simulink model "NarwhaleSimscape"  (R2021b)
settings: Solver=VariableStepAuto  StartTime=0.0  StopTime=12  FixedStep=10^-3  RelTol=1e-3
undefined symbols (not defined in the file): X, Y, Z
libraries: nesl_utility x34, sm_lib x28, slpidlib x5
(part 3 of 3)

== matlab function NarwhaleSimscape/NarWhale/IVK_5chi_dot ==
  data: q input; qv output; chi_dot input
function qv = IVK(q,chi_dot) %q,qv5,chi_dot  % q,taskspace
% h1= 275.99/1000; % lasted
% h2= 380/1000;
% l1= 20.01/1000;
% l2= 380/1000;
% l3= 235/1000;
% h1= 275.99/1000; % lasted
h2= 380/1000;
l1= 20/1000;
l2= 380/1000;
l3= 268.23/1000;

% qv = [                                                                                                                                                                                                                                                                                                                                                                                                                                                                                                                                                                                                                                                                                                                                                                                                                                                                                                                                                                                                                                                                                                                                                                                                                                                                                                                                                                                                                                                                                                                                                                                                                                                                                                                                                                                                                                                                                                                                                                                                                                                                                                                                                                                                                                                                                                                                                                                                                                                                                                                                                                                                                                                                                                                                                                                                                                                                                                                                                                                                                                                                                                                                                                                                                                                                                                                                                                                                                                                                                                                                                                                                                                                                                                                                                                                                                                                                                                                                                                                                                                                                                                                                                                                                                                                                                                                                                                                                                                                                                                                                                                                                                                                                                                                                                                                                                                                                                                                                                                                                                                                                                                                                                                                                                                                                                                                                                                                                                                                                                                                                                                                                                                                                                                                                                                                                                                                                                                                                                                                                                                                                                                                                                                                                                                                                                                                                                                                                                                                                                                                                                                                                                                                                                       (taskspace(4)*cos(q(1)) - taskspace(3)*sin(q(1)))/(l1 + l2*cos(q(2) + q(3)) - 1.0*h2*sin(q(2)) + l3*sin(q(2) + q(3) + q(4)));
%                                                                                                                                                                                                                                                                                                                                                                                                                                                                                                                                                                                                                                                                                                                                                                                                                                                                                                                                                                                                                                                                                                                                                                                                                                                                                                                                                                                                                                                                                                                                                                                                                                                                                                                                                                                                                                                                                                                                                                                                                                                                                                                                                                                                                                                                                                                                                                                                                                                                                                                                                                                                                                                                                                                                                                                                                                                                                                                                                                                                                                                                                                                                                                     -(1.0*(l3^2*taskspace(2)*sin(q(2) + q(3) + q(4))^3*sin(q(2) + q(3))*sin(q(1))^3 + l1*taskspace(3)*cos(q(2) + q(3) + q(4))*cos(q(2) + q(3))*cos(q(1))^2 + l1*taskspace(5)*cos(q(2) + q(3) + q(4))*sin(q(2) + q(3))*cos(q(1))^3 + l2*taskspace(3)*cos(q(2) + q(3) + q(4))*cos(q(2) + q(3))^2*cos(q(1))^2 + l3*taskspace(3)*sin(q(2) + q(3) + q(4))^2*sin(q(2) + q(3))*sin(q(1))^2 + l1*l3*taskspace(1)*cos(q(2) + q(3) + q(4))^2*cos(q(2) + q(3))*sin(q(1))^2 - h2*taskspace(3)*cos(q(2) + q(3) + q(4))*cos(q(2) + q(3))*cos(q(1))^2*sin(q(2)) + l2*taskspace(4)*cos(q(2) + q(3) + q(4))*cos(q(2) + q(3))^2*cos(q(1))*sin(q(1)) + l3^2*taskspace(1)*cos(q(2) + q(3) + q(4))^2*sin(q(2) + q(3) + q(4))*cos(q(2) + q(3))*cos(q(1))^2 - h2*taskspace(5)*cos(q(2) + q(3) + q(4))*sin(q(2) + q(3))*cos(q(1))^3*sin(q(2)) + l1*taskspace(5)*cos(q(2) + q(3) + q(4))*sin(q(2) + q(3))*cos(q(1))*sin(q(1))^2 + l3^2*taskspace(1)*cos(q(2) + q(3) + q(4))*sin(q(2) + q(3) + q(4))^2*sin(q(2) + q(3))*cos(q(1))^2 + l3^2*taskspace(1)*cos(q(2) + q(3) + q(4))^2*sin(q(2) + q(3) + q(4))*cos(q(2) + q(3))*sin(q(1))^2 + l3^2*taskspace(2)*cos(q(2) + q(3) + q(4))*sin(q(2) + q(3) + q(4))^2*cos(q(2) + q(3))*sin(q(1))^3 + l1*l3*taskspace(2)*sin(q(2) + q(3) + q(4))^2*sin(q(2) + q(3))*sin(q(1))^3 - l3*taskspace(4)*sin(q(2) + q(3) + q(4))^2*sin(q(2) + q(3))*cos(q(1))*sin(q(1)) + l3^2*taskspace(1)*cos(q(2) + q(3) + q(4))*sin(q(2) + q(3) + q(4))^2*sin(q(2) + q(3))*sin(q(1))^2 + l3*taskspace(3)*cos(q(2) + q(3) + q(4))*sin(q(2) + q(3) + q(4))*cos(q(2) + q(3))*cos(q(1))^2 + l2*l3*taskspace(1)*cos(q(2) + q(3) + q(4))^2*cos(q(2) + q(3))^2*cos(q(1))^2 + l3*taskspace(3)*cos(q(2) + q(3) + q(4))*sin(q(2) + q(3) + q(4))*cos(q(2) + q(3))*sin(q(1))^2 + l3*taskspace(5)*cos(q(2) + q(3) + q(4))*sin(q(2) + q(3) + q(4))*sin(q(2) + q(3))*cos(q(1))^3 + l2*l3*taskspace(1)*cos(q(2) + q(3) + q(4))^2*cos(q(2) + q(3))^2*sin(q(1))^2 + l1*taskspace(4)*cos(q(2) + q(3) + q(4))*cos(q(2) + q(3))*cos(q(1))*sin(q(1)) + l2*taskspace(5)*cos(q(2) + q(3) + q(4))*cos(q(2) + q(3))*sin(q(2) + q(3))*cos(q(1))^3 + l3^2*taskspace(2)*sin(q(2) + q(3) + q(4))^3*sin(q(2) + q(3))*cos(q(1))^2*sin(q(1)) + l1*l3*taskspace(1)*cos(q(2) + q(3) + q(4))^2*cos(q(2) + q(3))*cos(q(1))^2 + l1*l3*taskspace(2)*sin(q(2) + q(3) + q(4))^2*sin(q(2) + q(3))*cos(q(1))^2*sin(q(1)) - h2*taskspace(5)*cos(q(2) + q(3) + q(4))*sin(q(2) + q(3))*cos(q(1))*sin(q(1))^2*sin(q(2)) - h2*l3*taskspace(2)*sin(q(2) + q(3) + q(4))^2*sin(q(2) + q(3))*sin(q(1))^3*sin(q(2)) + l2*l3*taskspace(2)*cos(q(2) + q(3) + q(4))*sin(q(2) + q(3) + q(4))*cos(q(2) + q(3))^2*sin(q(1))^3 + l3*taskspace(5)*cos(q(2) + q(3) + q(4))*sin(q(2) + q(3) + q(4))*sin(q(2) + q(3))*cos(q(1))*sin(q(1))^2 - h2*taskspace(4)*cos(q(2) + q(3) + q(4))*cos(q(2) + q(3))*cos(q(1))*sin(q(1))*sin(q(2)) + l2*taskspace(5)*cos(q(2) + q(3) + q(4))*cos(q(2) + q(3))*sin(q(2) + q(3))*cos(q(1))*sin(q(1))^2 + l2*l3*taskspace(2)*sin(q(2) + q(3) + q(4))^2*cos(q(2) + q(3))*sin(q(2) + q(3))*sin(q(1))^3 + l1*l3*taskspace(1)*cos(q(2) + q(3) + q(4))*sin(q(2) + q(3) + q(4))*sin(q(2) + q(3))*cos(q(1))^2 + l1*l3*taskspace(2)*cos(q(2) + q(3) + q(4))*sin(q(2) + q(3) + q(4))*cos(q(2) + q(3))*sin(q(1))^3 - h2*l3*taskspace(1)*cos(q(2) + q(3) + q(4))^2*cos(q(2) + q(3))*cos(q(1))^2*sin(q(2)) + l1*l3*taskspace(1)*cos(q(2) + q(3) + q(4))*sin(q(2) + q(3) + q(4))*sin(q(2) + q(3))*sin(q(1))^2 - h2*l3*taskspace(1)*cos(q(2) + q(3) + q(4))^2*cos(q(2) + q(3))*sin(q(1))^2*sin(q(2)) + l3^2*taskspace(2)*cos(q(2) + q(3) + q(4))*sin(q(2) + q(3) + q(4))^2*cos(q(2) + q(3))*cos(q(1))^2*sin(q(1)) + l2*l3*taskspace(2)*cos(q(2) + q(3) + q(4))*sin(q(2) + q(3) + q(4))*cos(q(2) + q(3))^2*cos(q(1))^2*sin(q(1)) + l2*l3*taskspace(1)*cos(q(2) + q(3) + q(4))*sin(q(2) + q(3) + q(4))*cos(q(2) + q(3))*sin(q(2) + q(3))*cos(q(1))^2 + l2*l3*taskspace(1)*cos(q(2) + q(3) + q(4))*sin(q(2) + q(3) + q(4))*cos(q(2) + q(3))*sin(q(2) + q(3))*sin(q(1))^2 + l2*l3*taskspace(2)*sin(q(2) + q(3) + q(4))^2*cos(q(2) + q(3))*sin(q(2) + q(3))*cos(q(1))^2*sin(q(1)) + l1*l3*taskspace(2)*cos(q(2) + q(3) + q(4))*sin(q(2) + q(3) + q(4))*cos(q(2) + q(3))*cos(q(1))^2*sin(q(1)) - h2*l3*taskspace(1)*cos(q(2) + q(3) + q(4))*sin(q(2) + q(3) + q(4))*sin(q(2) + q(3))*cos(q(1))^2*sin(q(2)) - h2*l3*taskspace(2)*cos(q(2) + q(3) + q(4))*sin(q(2) + q(3) + q(4))*cos(q(2) + q(3))*sin(q(1))^3*sin(q(2)) - h2*l3*taskspace(1)*cos(q(2) + q(3) + q(4))*sin(q(2) + q(3) + q(4))*sin(q(2) + q(3))*sin(q(1))^2*sin(q(2)) - h2*l3*taskspace(2)*sin(q(2) + q(3) + q(4))^2*sin(q(2) + q(3))*cos(q(1))^2*sin(q(1))*sin(q(2)) - h2*l3*taskspace(2)*cos(q(2) + q(3) + q(4))*sin(q(2) + q(3) + q(4))*cos(q(2) + q(3))*cos(q(1))^2*sin(q(1))*sin(q(2))))/(h2*cos(q(1))*cos(q(3))*(0.5*l3*sin(2*q(2) + 2*q(3) + 2*q(4)) + 0.5*l2*cos(2.0*q(2) + 2.0*q(3) + q(4)) + 0.5*h2*sin(q(3) + q(4)) - 0.5*h2*sin(2.0*q(2) + q(3) + q(4)) + 0.5*l2*cos(q(4)) + l1*cos(q(2) + q(3) + q(4))));
% (1.0*(h2^2*taskspace(3)*cos(q(2) + q(3) + q(4))*cos(q(1))^2*sin(q(2))^2 + l2^2*taskspace(3)*cos(q(2) + q(3) + q(4))*cos(q(2) + q(3))^2*cos(q(1))^2 + h2^2*l3*taskspace(1)*cos(q(2) + q(3) + q(4))^2*sin(q(1))^2*sin(q(2))^2 + l2*l3*taskspace(3)*sin(q(2) + q(3) + q(4))^2*sin(q(2) + q(3))*sin(q(1))^2 + l2^2*taskspace(5)*cos(q(2) + q(3) + q(4))*cos(q(2) + q(3))*sin(q(2) + q(3))*cos(q(1))^3 + h2*l3*taskspace(3)*sin(q(2) + q(3) + q(4))^2*cos(q(2))*sin(q(1))^2 + l2^2*taskspace(4)*cos(q(2) + q(3) + q(4))*cos(q(2) + q(3))^2*cos(q(1))*sin(q(1)) + l2*l3^2*taskspace(2)*sin(q(2) + q(3) + q(4))^3*sin(q(2) + q(3))*sin(q(1))^3 + l1*l2*taskspace(3)*cos(q(2) + q(3) + q(4))*cos(q(2) + q(3))*cos(q(1))^2 - 1.0*h2^2*taskspace(5)*cos(q(2) + q(3) + q(4))*cos(q(1))^3*cos(q(2))*sin(q(2)) + h2*l3^2*taskspace(2)*sin(q(2) + q(3) + q(4))^3*cos(q(2))*sin(q(1))^3 + l1*l2*taskspace(5)*cos(q(2) + q(3) + q(4))*sin(q(2) + q(3))*cos(q(1))^3 + h2^2*taskspace(4)*cos(q(2) + q(3) + q(4))*cos(q(1))*sin(q(1))*sin(q(2))^2 + l2^2*l3*taskspace(1)*cos(q(2) + q(3) + q(4))^2*cos(q(2) + q(3))^2*cos(q(1))^2 + h2*l1*taskspace(5)*cos(q(2) + q(3) + q(4))*cos(q(1))^3*cos(q(2)) + l2^2*l3*taskspace(1)*cos(q(2) + q(3) + q(4))^2*cos(q(2) + q(3))^2*sin(q(1))^2 - 1.0*h2*l1*taskspace(3)*cos(q(2) + q(3) + q(4))*cos(q(1))^2*sin(q(2)) + h2^2*l3*taskspace(1)*cos(q(2) + q(3) + q(4))^2*cos(q(1))^2*sin(q(2))^2 - 1.0*h2*l3*taskspace(3)*cos(q(2) + q(3) + q(4))*sin(q(2) + q(3) + q(4))*sin(q(1))^2*sin(q(2)) + l1*l2*taskspace(4)*cos(q(2) + q(3) + q(4))*cos(q(2) + q(3))*cos(q(1))*sin(q(1)) + l2^2*taskspace(5)*cos(q(2) + q(3) + q(4))*cos(q(2) + q(3))*sin(q(2) + q(3))*cos(q(1))*sin(q(1))^2 + l2^2*l3*taskspace(2)*sin(q(2) + q(3) + q(4))^2*cos(q(2) + q(3))*sin(q(2) + q(3))*sin(q(1))^3 - 1.0*h2*l1*taskspace(4)*cos(q(2) + q(3) + q(4))*cos(q(1))*sin(q(1))*sin(q(2)) + l2*l3^2*taskspace(2)*sin(q(2) + q(3) + q(4))^3*sin(q(2) + q(3))*cos(q(1))^2*sin(q(1)) + l1*l2*l3*taskspace(1)*cos(q(2) + q(3) + q(4))^2*cos(q(2) + q(3))*cos(q(1))^2 + h2*l2*taskspace(5)*cos(q(2) + q(3) + q(4))*cos(q(2) + q(3))*cos(q(1))^3*cos(q(2)) + l1*l2*l3*taskspace(1)*cos(q(2) + q(3) + q(4))^2*cos(q(2) + q(3))*sin(q(1))^2 + h2*l3^2*taskspace(2)*sin(q(2) + q(3) + q(4))^3*cos(q(1))^2*cos(q(2))*sin(q(1)) - 2.0*h2*l2*taskspace(3)*cos(q(2) + q(3) + q(4))*cos(q(2) + q(3))*cos(q(1))^2*sin(q(2)) + l2*l3^2*taskspace(1)*cos(q(2) + q(3) + q(4))^2*sin(q(2) + q(3) + q(4))*cos(q(2) + q(3))*cos(q(1))^2 - 1.0*h2^2*taskspace(5)*cos(q(2) + q(3) + q(4))*cos(q(1))*cos(q(2))*sin(q(1))^2*sin(q(2)) - 1.0*h2^2*l3*taskspace(2)*sin(q(2) + q(3) + q(4))^2*cos(q(2))*sin(q(1))^3*sin(q(2)) - 1.0*h2*l2*taskspace(5)*cos(q(2) + q(3) + q(4))*sin(q(2) + q(3))*cos(q(1))^3*sin(q(2)) + l1*l2*taskspace(5)*cos(q(2) + q(3) + q(4))*sin(q(2) + q(3))*cos(q(1))*sin(q(1))^2 + l2*l3^2*taskspace(1)*cos(q(2) + q(3) + q(4))*sin(q(2) + q(3) + q(4))^2*sin(q(2) + q(3))*cos(q(1))^2 + l2*l3^2*taskspace(1)*cos(q(2) + q(3) + q(4))^2*sin(q(2) + q(3) + q(4))*cos(q(2) + q(3))*sin(q(1))^2 + l2*l3^2*taskspace(2)*cos(q(2) + q(3) + q(4))*sin(q(2) + q(3) + q(4))^2*cos(q(2) + q(3))*sin(q(1))^3 + l2^2*l3*taskspace(2)*cos(q(2) + q(3) + q(4))*sin(q(2) + q(3) + q(4))*cos(q(2) + q(3))^2*sin(q(1))^3 + l1*l2*l3*taskspace(2)*sin(q(2) + q(3) + q(4))^2*sin(q(2) + q(3))*sin(q(1))^3 - 1.0*l2*l3*taskspace(4)*sin(q(2) + q(3) + q(4))^2*sin(q(2) + q(3))*cos(q(1))*sin(q(1)) + l2*l3^2*taskspace(1)*cos(q(2) + q(3) + q(4))*sin(q(2) + q(3) + q(4))^2*sin(q(2) + q(3))*sin(q(1))^2 - 1.0*h2*l1*l3*taskspace(1)*cos(q(2) + q(3) + q(4))^2*cos(q(1))^2*sin(q(2)) + h2*l1*taskspace(5)*cos(q(2) + q(3) + q(4))*cos(q(1))*cos(q(2))*sin(q(1))^2 + h2*l3^2*taskspace(1)*cos(q(2) + q(3) + q(4))*sin(q(2) + q(3) + q(4))^2*cos(q(1))^2*cos(q(2)) - 1.0*h2*l1*l3*taskspace(1)*cos(q(2) + q(3) + q(4))^2*sin(q(1))^2*sin(q(2)) + h2*l1*l3*taskspace(2)*sin(q(2) + q(3) + q(4))^2*cos(q(2))*sin(q(1))^3 - 1.0*h2*l3*taskspace(4)*sin(q(2) + q(3) + q(4))^2*cos(q(1))*cos(q(2))*sin(q(1)) + h2*l3^2*taskspace(1)*cos(q(2) + q(3) + q(4))*sin(q(2) + q(3) + q(4))^2*cos(q(2))*sin(q(1))^2 - 1.0*h2*l3^2*taskspace(1)*cos(q(2) + q(3) + q(4))^2*sin(q(2) + q(3) + q(4))*cos(q(1))^2*sin(q(2)) + l2*l3*taskspace(3)*cos(q(2) + q(3) + q(4))*sin(q(2) + q(3) + q(4))*cos(q(2) + q(3))*cos(q(1))^2 - 1.0*h2*l3^2*taskspace(1)*cos(q(2) + q(3) + q(4))^2*sin(q(2) + q(3) + q(4))*sin(q(1))^2*sin(q(2)) - 1.0*h2*l3^2*taskspace(2)*cos(q(2) + q(3) + q(4))*sin(q(2) + q(3) + q(4))^2*sin(q(1))^3*sin(q(2)) + h2^2*l3*taskspace(2)*cos(q(2) + q(3) + q(4))*sin(q(2) + q(3) + q(4))*sin(q(1))^3*sin(q(2))^2 + l2*l3*taskspace(3)*cos(q(2) + q(3) + q(4))*sin(q(2) + q(3) + q(4))*cos(q(2) + q(3))*sin(q(1))^2 + l2*l3*taskspace(5)*cos(q(2) + q(3) + q(4))*sin(q(2) + q(3) + q(4))*sin(q(2) + q(3))*cos(q(1))^3 + h2*l3*taskspace(5)*cos(q(2) + q(3) + q(4))*sin(q(2) + q(3) + q(4))*cos(q(1))^3*cos(q(2)) - 1.0*h2*l3*taskspace(3)*cos(q(2) + q(3) + q(4))*sin(q(2) + q(3) + q(4))*cos(q(1))^2*sin(q(2)) - 2.0*h2*l2*taskspace(4)*cos(q(2) + q(3) + q(4))*cos(q(2) + q(3))*cos(q(1))*sin(q(1))*sin(q(2)) + l2^2*l3*taskspace(2)*sin(q(2) + q(3) + q(4))^2*cos(q(2) + q(3))*sin(q(2) + q(3))*cos(q(1))^2*sin(q(1)) - 1.0*h2^2*l3*taskspace(1)*cos(q(2) + q(3) + q(4))*sin(q(2) + q(3) + q(4))*cos(q(1))^2*cos(q(2))*sin(q(2)) + l1*l2*l3*taskspace(1)*cos(q(2) + q(3) + q(4))*sin(q(2) + q(3) + q(4))*sin(q(2) + q(3))*cos(q(1))^2 + l1*l2*l3*taskspace(2)*cos(q(2) + q(3) + q(4))*sin(q(2) + q(3) + q(4))*cos(q(2) + q(3))*sin(q(1))^3 - 1.0*h2^2*l3*taskspace(1)*cos(q(2) + q(3) + q(4))*sin(q(2) + q(3) + q(4))*cos(q(2))*sin(q(1))^2*sin(q(2)) - 2.0*h2*l2*l3*taskspace(1)*cos(q(2) + q(3) + q(4))^2*cos(q(2) + q(3))*cos(q(1))^2*sin(q(2)) + l1*l2*l3*taskspace(1)*cos(q(2) + q(3) + q(4))*sin(q(2) + q(3) + q(4))*sin(q(2) + q(3))*sin(q(1))^2 + h2*l2*taskspace(5)*cos(q(2) + q(3) + q(4))*cos(q(2) + q(3))*cos(q(1))*cos(q(2))*sin(q(1))^2 - 2.0*h2*l2*l3*taskspace(1)*cos(q(2) + q(3) + q(4))^2*cos(q(2) + q(3))*sin(q(1))^2*sin(q(2)) + h2*l2*l3*taskspace(2)*sin(q(2) + q(3) + q(4))^2*cos(q(2) + q(3))*cos(q(2))*sin(q(1))^3 + h2*l1*l3*taskspace(1)*cos(q(2) + q(3) + q(4))*sin(q(2) + q(3) + q(4))*cos(q(1))^2*cos(q(2)) - 1.0*h2^2*l3*taskspace(2)*sin(q(2) + q(3) + q(4))^2*cos(q(1))^2*cos(q(2))*sin(q(1))*sin(q(2)) + l2*l3^2*taskspace(2)*cos(q(2) + q(3) + q(4))*sin(q(2) + q(3) + q(4))^2*cos(q(2) + q(3))*cos(q(1))^2*sin(q(1)) + l2^2*l3*taskspace(2)*cos(q(2) + q(3) + q(4))*sin(q(2) + q(3) + q(4))*cos(q(2) + q(3))^2*cos(q(1))^2*sin(q(1)) + h2*l1*l3*taskspace(1)*cos(q(2) + q(3) + q(4))*sin(q(2) + q(3) + q(4))*cos(q(2))*sin(q(1))^2 + l1*l2*l3*taskspace(2)*sin(q(2) + q(3) + q(4))^2*sin(q(2) + q(3))*cos(q(1))^2*sin(q(1)) - 1.0*h2*l2*taskspace(5)*cos(q(2) + q(3) + q(4))*sin(q(2) + q(3))*cos(q(1))*sin(q(1))^2*sin(q(2)) - 1.0*h2*l2*l3*taskspace(2)*sin(q(2) + q(3) + q(4))^2*sin(q(2) + q(3))*sin(q(1))^3*sin(q(2)) - 1.0*h2*l1*l3*taskspace(2)*cos(q(2) + q(3) + q(4))*sin(q(2) + q(3) + q(4))*sin(q(1))^3*sin(q(2)) + h2*l1*l3*taskspace(2)*sin(q(2) + q(3) + q(4))^2*cos(q(1))^2*cos(q(2))*sin(q(1)) - 1.0*h2*l3^2*taskspace(2)*cos(q(2) + q(3) + q(4))*sin(q(2) + q(3) + q(4))^2*cos(q(1))^2*sin(q(1))*sin(q(2)) + h2^2*l3*taskspace(2)*cos(q(2) + q(3) + q(4))*sin(q(2) + q(3) + q(4))*cos(q(1))^2*sin(q(1))*sin(q(2))^2 + l2*l3*taskspace(5)*cos(q(2) + q(3) + q(4))*sin(q(2) + q(3) + q(4))*sin(q(2) + q(3))*cos(q(1))*sin(q(1))^2 + h2*l3*taskspace(5)*cos(q(2) + q(3) + q(4))*sin(q(2) + q(3) + q(4))*cos(q(1))*cos(q(2))*sin(q(1))^2 + l2^2*l3*taskspace(1)*cos(q(2) + q(3) + q(4))*sin(q(2) + q(3) + q(4))*cos(q(2) + q(3))*sin(q(2) + q(3))*cos(q(1))^2 + l2^2*l3*taskspace(1)*cos(q(2) + q(3) + q(4))*sin(q(2) + q(3) + q(4))*cos(q(2) + q(3))*sin(q(2) + q(3))*sin(q(1))^2 + h2*l2*l3*taskspace(1)*cos(q(2) + q(3) + q(4))*sin(q(2) + q(3) + q(4))*cos(q(2) + q(3))*cos(q(2))*sin(q(1))^2 + l1*l2*l3*taskspace(2)*cos(q(2) + q(3) + q(4))*sin(q(2) + q(3) + q(4))*cos(q(2) + q(3))*cos(q(1))^2*sin(q(1)) - 1.0*h2*l2*l3*taskspace(1)*cos(q(2) + q(3) + q(4))*sin(q(2) + q(3) + q(4))*sin(q(2) + q(3))*cos(q(1))^2*sin(q(2)) - 2.0*h2*l2*l3*taskspace(2)*cos(q(2) + q(3) + q(4))*sin(q(2) + q(3) + q(4))*cos(q(2) + q(3))*sin(q(1))^3*sin(q(2)) + h2*l2*l3*taskspace(2)*sin(q(2) + q(3) + q(4))^2*cos(q(2) + q(3))*cos(q(1))^2*cos(q(2))*sin(q(1)) - 1.0*h2*l2*l3*taskspace(1)*cos(q(2) + q(3) + q(4))*sin(q(2) + q(3) + q(4))*sin(q(2) + q(3))*sin(q(1))^2*sin(q(2)) - 1.0*h2*l2*l3*taskspace(2)*sin(q(2) + q(3) + q(4))^2*sin(q(2) + q(3))*cos(q(1))^2*sin(q(1))*sin(q(2)) - 1.0*h2*l1*l3*taskspace(2)*cos(q(2) + q(3) + q(4))*sin(q(2) + q(3) + q(4))*cos(q(1))^2*sin(q(1))*sin(q(2)) + h2*l2*l3*taskspace(1)*cos(q(2) + q(3) + q(4))*sin(q(2) + q(3) + q(4))*cos(q(2) + q(3))*cos(q(1))^2*cos(q(2)) - 2.0*h2*l2*l3*taskspace(2)*cos(q(2) + q(3) + q(4))*sin(q(2) + q(3) + q(4))*cos(q(2) + q(3))*cos(q(1))^2*sin(q(1))*sin(q(2))))/(h2*l2*cos(q(1))*cos(q(3))*(0.5*l3*sin(2*q(2) + 2*q(3) + 2*q(4)) + 0.5*l2*cos(2.0*q(2) + 2.0*q(3) + q(4)) + 0.5*h2*sin(q(3) + q(4)) - 0.5*h2*sin(2.0*q(2) + q(3) + q(4)) + 0.5*l2*cos(q(4)) + l1*cos(q(2) + q(3) + q(4))));
%                                                                                                                                                                                                                                                                                                                                                                                                                                                                                                                                                                                                                                                                                                                                                                                                                                                                                                                                                                                                                                                                                                                                                                                     -(1.0*(l3^2*taskspace(2)*sin(q(2) + q(3) + q(4))^3*cos(q(2))*sin(q(1))^3 + l1*taskspace(5)*cos(q(2) + q(3) + q(4))*cos(q(1))^3*cos(q(2)) - l1*taskspace(3)*cos(q(2) + q(3) + q(4))*cos(q(1))^2*sin(q(2)) + h2*taskspace(3)*cos(q(2) + q(3) + q(4))*cos(q(1))^2*sin(q(2))^2 + l3*taskspace(3)*sin(q(2) + q(3) + q(4))^2*cos(q(2))*sin(q(1))^2 + l2*taskspace(5)*cos(q(2) + q(3) + q(4))*cos(q(2) + q(3))*cos(q(1))^3*cos(q(2)) + l3^2*taskspace(2)*sin(q(2) + q(3) + q(4))^3*cos(q(1))^2*cos(q(2))*sin(q(1)) - l2*taskspace(3)*cos(q(2) + q(3) + q(4))*cos(q(2) + q(3))*cos(q(1))^2*sin(q(2)) + l2*taskspace(3)*sin(q(2) + q(3) + q(4))*cos(q(2) + q(3))*cos(q(2))*sin(q(1))^2 - l1*l3*taskspace(1)*cos(q(2) + q(3) + q(4))^2*cos(q(1))^2*sin(q(2)) - h2*taskspace(5)*cos(q(2) + q(3) + q(4))*cos(q(1))^3*cos(q(2))*sin(q(2)) + l1*taskspace(5)*cos(q(2) + q(3) + q(4))*cos(q(1))*cos(q(2))*sin(q(1))^2 + l2*taskspace(3)*sin(q(2) + q(3) + q(4))*sin(q(2) + q(3))*sin(q(1))^2*sin(q(2)) + l3^2*taskspace(1)*cos(q(2) + q(3) + q(4))*sin(q(2) + q(3) + q(4))^2*cos(q(1))^2*cos(q(2)) - l1*l3*taskspace(1)*cos(q(2) + q(3) + q(4))^2*sin(q(1))^2*sin(q(2)) + l1*l3*taskspace(2)*sin(q(2) + q(3) + q(4))^2*cos(q(2))*sin(q(1))^3 + h2*taskspace(4)*cos(q(2) + q(3) + q(4))*cos(q(1))*sin(q(1))*sin(q(2))^2 - l3*taskspace(4)*sin(q(2) + q(3) + q(4))^2*cos(q(1))*cos(q(2))*sin(q(1)) + l3^2*taskspace(1)*cos(q(2) + q(3) + q(4))*sin(q(2) + q(3) + q(4))^2*cos(q(2))*sin(q(1))^2 - l3^2*taskspace(1)*cos(q(2) + q(3) + q(4))^2*sin(q(2) + q(3) + q(4))*cos(q(1))^2*sin(q(2)) - l3^2*taskspace(1)*cos(q(2) + q(3) + q(4))^2*sin(q(2) + q(3) + q(4))*sin(q(1))^2*sin(q(2)) - l3^2*taskspace(2)*cos(q(2) + q(3) + q(4))*sin(q(2) + q(3) + q(4))^2*sin(q(1))^3*sin(q(2)) + l3*taskspace(5)*cos(q(2) + q(3) + q(4))*sin(q(2) + q(3) + q(4))*cos(q(1))^3*cos(q(2)) - l3*taskspace(3)*cos(q(2) + q(3) + q(4))*sin(q(2) + q(3) + q(4))*cos(q(1))^2*sin(q(2)) + h2*l3*taskspace(1)*cos(q(2) + q(3) + q(4))^2*cos(q(1))^2*sin(q(2))^2 - l3*taskspace(3)*cos(q(2) + q(3) + q(4))*sin(q(2) + q(3) + q(4))*sin(q(1))^2*sin(q(2)) + h2*l3*taskspace(1)*cos(q(2) + q(3) + q(4))^2*sin(q(1))^2*sin(q(2))^2 + l2^2*taskspace(1)*cos(q(2) + q(3) + q(4))*cos(q(2) + q(3))^2*cos(q(1))^2*cos(q(2)) + l2^2*taskspace(1)*cos(q(2) + q(3) + q(4))*cos(q(2) + q(3))^2*cos(q(2))*sin(q(1))^2 + l2^2*taskspace(2)*sin(q(2) + q(3) + q(4))*cos(q(2) + q(3))^2*cos(q(2))*sin(q(1))^3 - l1*taskspace(4)*cos(q(2) + q(3) + q(4))*cos(q(1))*sin(q(1))*sin(q(2)) + l1*l3*taskspace(1)*cos(q(2) + q(3) + q(4))*sin(q(2) + q(3) + q(4))*cos(q(2))*sin(q(1))^2 - h2*l2*taskspace(2)*sin(q(2) + q(3) + q(4))*sin(q(2) + q(3))*sin(q(1))^3*sin(q(2))^2 + l2*l3*taskspace(2)*sin(q(2) + q(3) + q(4))^2*sin(q(2) + q(3))*sin(q(1))^3*sin(q(2)) - l1*l3*taskspace(2)*cos(q(2) + q(3) + q(4))*sin(q(2) + q(3) + q(4))*sin(q(1))^3*sin(q(2)) + l1*l3*taskspace(2)*sin(q(2) + q(3) + q(4))^2*cos(q(1))^2*cos(q(2))*sin(q(1)) - h2*taskspace(5)*cos(q(2) + q(3) + q(4))*cos(q(1))*cos(q(2))*sin(q(1))^2*sin(q(2)) + l2^2*taskspace(1)*cos(q(2) + q(3) + q(4))*cos(q(2) + q(3))*sin(q(2) + q(3))*cos(q(1))^2*sin(q(2)) - h2*l3*taskspace(2)*sin(q(2) + q(3) + q(4))^2*cos(q(2))*sin(q(1))^3*sin(q(2)) + l2^2*taskspace(1)*cos(q(2) + q(3) + q(4))*cos(q(2) + q(3))*sin(q(2) + q(3))*sin(q(1))^2*sin(q(2)) - l3^2*taskspace(2)*cos(q(2) + q(3) + q(4))*sin(q(2) + q(3) + q(4))^2*cos(q(1))^2*sin(q(1))*sin(q(2)) + l2^2*taskspace(2)*sin(q(2) + q(3) + q(4))*cos(q(2) + q(3))*sin(q(2) + q(3))*sin(q(1))^3*sin(q(2)) + l3*taskspace(5)*cos(q(2) + q(3) + q(4))*sin(q(2) + q(3) + q(4))*cos(q(1))*cos(q(2))*sin(q(1))^2 + h2*l3*taskspace(2)*cos(q(2) + q(3) + q(4))*sin(q(2) + q(3) + q(4))*sin(q(1))^3*sin(q(2))^2 + l1*l2*taskspace(1)*cos(q(2) + q(3) + q(4))*cos(q(2) + q(3))*cos(q(1))^2*cos(q(2)) + l1*l2*taskspace(1)*cos(q(2) + q(3) + q(4))*cos(q(2) + q(3))*cos(q(2))*sin(q(1))^2 + l1*l2*taskspace(1)*cos(q(2) + q(3) + q(4))*sin(q(2) + q(3))*cos(q(1))^2*sin(q(2)) + l1*l2*taskspace(2)*sin(q(2) + q(3) + q(4))*cos(q(2) + q(3))*cos(q(2))*sin(q(1))^3 - l2*taskspace(4)*cos(q(2) + q(3) + q(4))*cos(q(2) + q(3))*cos(q(1))*sin(q(1))*sin(q(2)) - l2*taskspace(4)*sin(q(2) + q(3) + q(4))*cos(q(2) + q(3))*cos(q(1))*cos(q(2))*sin(q(1)) + l1*l2*taskspace(1)*cos(q(2) + q(3) + q(4))*sin(q(2) + q(3))*sin(q(1))^2*sin(q(2)) + l1*l2*taskspace(2)*sin(q(2) + q(3) + q(4))*sin(q(2) + q(3))*sin(q(1))^3*sin(q(2)) + l2^2*taskspace(2)*sin(q(2) + q(3) + q(4))*cos(q(2) + q(3))^2*cos(q(1))^2*cos(q(2))*sin(q(1)) - l2*taskspace(4)*sin(q(2) + q(3) + q(4))*sin(q(2) + q(3))*cos(q(1))*sin(q(1))*sin(q(2)) - l2*l3*taskspace(1)*cos(q(2) + q(3) + q(4))^2*cos(q(2) + q(3))*cos(q(1))^2*sin(q(2)) + l2*taskspace(5)*cos(q(2) + q(3) + q(4))*cos(q(2) + q(3))*cos(q(1))*cos(q(2))*sin(q(1))^2 - h2*l2*taskspace(1)*cos(q(2) + q(3) + q(4))*sin(q(2) + q(3))*cos(q(1))^2*sin(q(2))^2 - l2*l3*taskspace(1)*cos(q(2) + q(3) + q(4))^2*cos(q(2) + q(3))*sin(q(1))^2*sin(q(2)) + 2.0*l2*l3*taskspace(2)*sin(q(2) + q(3) + q(4))^2*cos(q(2) + q(3))*cos(q(2))*sin(q(1))^3 + l1*l3*taskspace(1)*cos(q(2) + q(3) + q(4))*sin(q(2) + q(3) + q(4))*cos(q(1))^2*cos(q(2)) - h2*l2*taskspace(1)*cos(q(2) + q(3) + q(4))*sin(q(2) + q(3))*sin(q(1))^2*sin(q(2))^2 - h2*l3*taskspace(2)*sin(q(2) + q(3) + q(4))^2*cos(q(1))^2*cos(q(2))*sin(q(1))*sin(q(2)) + l2^2*taskspace(2)*sin(q(2) + q(3) + q(4))*cos(q(2) + q(3))*sin(q(2) + q(3))*cos(q(1))^2*sin(q(1))*sin(q(2)) + h2*l3*taskspace(2)*cos(q(2) + q(3) + q(4))*sin(q(2) + q(3) + q(4))*cos(q(1))^2*sin(q(1))*sin(q(2))^2 - h2*l2*taskspace(1)*cos(q(2) + q(3) + q(4))*cos(q(2) + q(3))*cos(q(1))^2*cos(q(2))*sin(q(2)) - h2*l2*taskspace(1)*cos(q(2) + q(3) + q(4))*cos(q(2) + q(3))*cos(q(2))*sin(q(1))^2*sin(q(2)) + l1*l2*taskspace(2)*sin(q(2) + q(3) + q(4))*cos(q(2) + q(3))*cos(q(1))^2*cos(q(2))*sin(q(1)) - h2*l2*taskspace(2)*sin(q(2) + q(3) + q(4))*cos(q(2) + q(3))*cos(q(2))*sin(q(1))^3*sin(q(2)) + l1*l2*taskspace(2)*sin(q(2) + q(3) + q(4))*sin(q(2) + q(3))*cos(q(1))^2*sin(q(1))*sin(q(2)) + 2.0*l2*l3*taskspace(1)*cos(q(2) + q(3) + q(4))*sin(q(2) + q(3) + q(4))*cos(q(2) + q(3))*cos(q(1))^2*cos(q(2)) + 2.0*l2*l3*taskspace(1)*cos(q(2) + q(3) + q(4))*sin(q(2) + q(3) + q(4))*cos(q(2) + q(3))*cos(q(2))*sin(q(1))^2 + l2*l3*taskspace(1)*cos(q(2) + q(3) + q(4))*sin(q(2) + q(3) + q(4))*sin(q(2) + q(3))*cos(q(1))^2*sin(q(2)) - l2*l3*taskspace(2)*cos(q(2) + q(3) + q(4))*sin(q(2) + q(3) + q(4))*cos(q(2) + q(3))*sin(q(1))^3*sin(q(2)) + 2.0*l2*l3*taskspace(2)*sin(q(2) + q(3) + q(4))^2*cos(q(2) + q(3))*cos(q(1))^2*cos(q(2))*sin(q(1)) + l2*l3*taskspace(1)*cos(q(2) + q(3) + q(4))*sin(q(2) + q(3) + q(4))*sin(q(2) + q(3))*sin(q(1))^2*sin(q(2)) - h2*l3*taskspace(1)*cos(q(2) + q(3) + q(4))*sin(q(2) + q(3) + q(4))*cos(q(1))^2*cos(q(2))*sin(q(2)) - h2*l2*taskspace(2)*sin(q(2) + q(3) + q(4))*sin(q(2) + q(3))*cos(q(1))^2*sin(q(1))*sin(q(2))^2 - h2*l3*taskspace(1)*cos(q(2) + q(3) + q(4))*sin(q(2) + q(3) + q(4))*cos(q(2))*sin(q(1))^2*sin(q(2)) + l2*l3*taskspace(2)*sin(q(2) + q(3) + q(4))^2*sin(q(2) + q(3))*cos(q(1))^2*sin(q(1))*sin(q(2)) - l1*l3*taskspace(2)*cos(q(2) + q(3) + q(4))*sin(q(2) + q(3) + q(4))*cos(q(1))^2*sin(q(1))*sin(q(2)) - h2*l2*taskspace(2)*sin(q(2) + q(3) + q(4))*cos(q(2) + q(3))*cos(q(1))^2*cos(q(2))*sin(q(1))*sin(q(2)) - l2*l3*taskspace(2)*cos(q(2) + q(3) + q(4))*sin(q(2) + q(3) + q(4))*cos(q(2) + q(3))*cos(q(1))^2*sin(q(1))*sin(q(2))))/(l2*cos(q(1))*cos(q(3))*(0.5*l3*sin(2*q(2) + 2*q(3) + 2*q(4)) + 0.5*l2*cos(2.0*q(2) + 2.0*q(3) + q(4)) + 0.5*h2*sin(q(3) + q(4)) - 0.5*h2*sin(2.0*q(2) + q(3) + q(4)) + 0.5*l2*cos(q(4)) + l1*cos(q(2) + q(3) + q(4))));
%                                                                                                                                                                                                                                                                                                                                                                                                                                                                                                                                                                                                                                                                                                                                                                                                                                                                                                                                                                                                                                                                                                                                                                                                                                                                                                                                                                                                                                                                                                                                                                                                                                                                                                                                                                                                                                                                                                                                                                                                                                                                                                                                                                                                                                                                                                                                                                                                                                                                                                                                                                                                                                                                                                                                                                                                                                                                                                                                                                                                                                                                                                                                                                                                                                                                                                                                                                                                                                                                                                                                                                                                                                                                                                                                                                                                                                                                                                                                                                                                                                                                                                                                                                                                                                                                                                                                                                                                                                                                                                                                                                                                                                                                                                                                                                                                                                                                                                                                                                                                                                                                                                                                                                                                                                                                                                                                                                                                                                                                                                                                                                                                                                                                                                                                                                                                                                                                                                                                                                                                                                                                                                                                                                                                                                                                                                                                                                                                                                                                                               -(1.0*(l1*taskspace(2) - 1.0*taskspace(4)*cos(q(1)) + taskspace(3)*sin(q(1)) - 1.0*h2*taskspace(2)*sin(q(2)) + 1.0*l3*taskspace(2)*sin(q(2) + q(3) + q(4)) + 1.0*l2*taskspace(2)*cos(q(2) + q(3))))/(0.5*l3*sin(2*q(2) + 2*q(3) + 2*q(4)) - 0.5*h2*sin(2*q(2) + q(3) + q(4)) + 0.5*h2*sin(q(3) + q(4)) + 0.5*l2*cos(q(4)) + 0.5*l2*cos(2*q(2) + 2*q(3) + q(4)) + 1.0*l1*cos(q(2) + q(3) + q(4)))]
%  
% 
%Jv5 ตรงแล้ว
% Jv5 =[ -sin(q(1))*(l1 + l2*cos(q(2) + q(3)) - h2*sin(q(2))), -cos(q(1))*(l2*sin(q(2) + q(3)) + h2*cos(q(2))), -l2*sin(q(2) + q(3))*cos(q(1));
%         cos(q(1))*(l1 + l2*cos(q(2) + q(3)) - h2*sin(q(2))), -sin(q(1))*(l2*sin(q(2) + q(3)) + h2*cos(q(2))), -l2*sin(q(2) + q(3))*sin(q(1));
%                                                   0,            l2*cos(q(2) + q(3)) - h2*sin(q(2)),          l2*cos(q(2) + q(3))]

% Jv52 = [                                                   1,                                               0,                              0,       -1;
%         -sin(q(1))*(l1 + l2*cos(q(2) + q(3)) - h2*sin(q(2))), -cos(q(1))*(l2*sin(q(2) + q(3)) + h2*cos(q(2))), -l2*sin(q(2) + q(3))*cos(q(1)),        0;
%          cos(q(1))*(l1 + l2*cos(q(2) + q(3)) - h2*sin(q(2))), -sin(q(1))*(l2*sin(q(2) + q(3)) + h2*cos(q(2))), -l2*sin(q(2) + q(3))*sin(q(1)),        0;
%                                                            0,              l2*cos(q(2) + q(3)) - h2*sin(q(2)),            l2*cos(q(2) + q(3)),        0]
%Jv52 ไม่ตรง
% Jev3 = [- sin(q(1))*(l1 + l2*cos(q(2) + q(3)) - h2*sin(q(2))) , l3*cos(q(1)) - cos(q(1))*(l2*sin(q(2) + q(3)) + h2*cos(q(2))), -cos(q(1))*(l2*sin(q(2) + q(3)) - l3);
%    cos(q(1))*(l1 + l2*cos(q(2) + q(3)) - h2*sin(q(2)))        , l3*sin(q(1)) - sin(q(1))*(l2*sin(q(2) + q(3)) + h2*cos(q(2))), -sin(q(1))*(l2*sin(q(2) + q(3)) - l3);
%                                                            0  ,  l2*cos(q(2) + q(3)) - h2*sin(q(2))                          ,  l2*cos(q(2) + q(3)) ];
%jev3 ไม่ถูก
% Jev4=[                                                     1,                                                             0,                                     0,                 -1;
%       - sin(q(1))*(l1 + l2*cos(q(2) + q(3)) - h2*sin(q(2))) , l3*cos(q(1)) - cos(q(1))*(l2*sin(q(2) + q(3)) + h2*cos(q(2))), -cos(q(1))*(l2*sin(q(2) + q(3)) - l3),                  0;
%         cos(q(1))*(l1 + l2*cos(q(2) + q(3)) - h2*sin(q(2))) , l3*sin(q(1)) - sin(q(1))*(l2*sin(q(2) + q(3)) + h2*cos(q(2))), -sin(q(1))*(l2*sin(q(2) + q(3)) - l3),                  0;
%                                                            0,                           l2*cos(q(2) + q(3)) - h2*sin(q(2)) ,                  l2*cos(q(2) + q(3)) ,                  0] 
% jev4 ไม่ตรงเลย
% q1 =q(1)
% q2=q(2)
% q3=q(3)
% q4 = -q2-q3
% Je =  [- sin(q1)*(l1 + l2*cos(q2 + q3) - h2*sin(q2)) - l3*sin(q2 + q3 + q4)*sin(q1), l3*cos(q2 + q3 + q4)*cos(q1) - cos(q1)*(l2*sin(q2 + q3) + h2*cos(q2)), -cos(q1)*(l2*sin(q2 + q3) - l3*cos(q2 + q3 + q4));
%   cos(q1)*(l1 + l2*cos(q2 + q3) - h2*sin(q2)) + l3*sin(q2 + q3 + q4)*cos(q1), l3*cos(q2 + q3 + q4)*sin(q1) - sin(q1)*(l2*sin(q2 + q3) + h2*cos(q2)), -sin(q1)*(l2*sin(q2 + q3) - l3*cos(q2 + q3 + q4));
%                                                                            0,                   l2*cos(q2 + q3) - h2*sin(q2) + l3*sin(q2 + q3 + q4),            l2*cos(q2 + q3) + l3*sin(q2 + q3 + q4)]
%  
% Je =[                                      0,                                      sin(q1),                        sin(q1),    sin(q1),  0;
%                                            0,                                     -cos(q1),                       -cos(q1),   -cos(q1),  0;
%                                            1,                                            0,                              0,          0, -1;
% -sin(q1)*(l1 + l2*cos(q2 + q3) - h2*sin(q2)), -cos(q1)*(l2*sin(q2 + q3) - l3 + h2*cos(q2)), cos(q1)*(l3 - l2*sin(q2 + q3)), l3*cos(q1),  0;
%  cos(q1)*(l1 + l2*cos(q2 + q3) - h2*sin(q2)), -sin(q1)*(l2*sin(q2 + q3) - l3 + h2*cos(q2)), sin(q1)*(l3 - l2*sin(q2 + q3)), l3*sin(q1),  0;
%                                            0,                 l2*cos(q2 + q3) - h2*sin(q2),                l2*cos(q2 + q3),          0,  0] 
q1=q(1)
q2=q(2)
q3=q(3)
q4=q(4)
q5=q(5)
inv_je =[                                                                                                                     0,  0,                                                         -sin(q1)/(l1*sin(q1)^2 + l1*cos(q1)^2 + l2*cos(q2 + q3)*cos(q1)^2 + l2*cos(q2 + q3)*sin(q1)^2 - h2*cos(q1)^2*sin(q2) - h2*sin(q1)^2*sin(q2)),                                                                cos(q1)/(l1*sin(q1)^2 + l1*cos(q1)^2 + l2*cos(q2 + q3)*cos(q1)^2 + l2*cos(q2 + q3)*sin(q1)^2 - h2*cos(q1)^2*sin(q2) - h2*sin(q1)^2*sin(q2)),                                                                                        0;
                                               -(l3*cos(q2 + q3))/(cos(q1)*(h2*cos(q2 + q3)*cos(q2) + h2*sin(q2 + q3)*sin(q2))),  0,                              -(cos(q2 + q3)*cos(q1))/(h2*cos(q2 + q3)*cos(q1)^2*cos(q2) + h2*cos(q2 + q3)*cos(q2)*sin(q1)^2 + h2*sin(q2 + q3)*cos(q1)^2*sin(q2) + h2*sin(q2 + q3)*sin(q1)^2*sin(q2)),                                    -(cos(q2 + q3)*sin(q1))/(h2*cos(q2 + q3)*cos(q1)^2*cos(q2) + h2*cos(q2 + q3)*cos(q2)*sin(q1)^2 + h2*sin(q2 + q3)*cos(q1)^2*sin(q2) + h2*sin(q2 + q3)*sin(q1)^2*sin(q2)),                        -sin(q2 + q3)/(h2*cos(q2 + q3)*cos(q2) + h2*sin(q2 + q3)*sin(q2));
                      -(h2*l3*sin(q2) - l2*l3*cos(q2 + q3))/(cos(q1)*(h2*l2*cos(q2 + q3)*cos(q2) + h2*l2*sin(q2 + q3)*sin(q2))),  0, (cos(q1)*(l2*cos(q2 + q3) - h2*sin(q2)))/(h2*l2*sin(q2 + q3)*cos(q1)^2*sin(q2) + h2*l2*sin(q2 + q3)*sin(q1)^2*sin(q2) + h2*l2*cos(q2 + q3)*cos(q1)^2*cos(q2) + h2*l2*cos(q2 + q3)*cos(q2)*sin(q1)^2), (l2*cos(q2 + q3)*sin(q1) - h2*sin(q1)*sin(q2))/(h2*l2*sin(q2 + q3)*cos(q1)^2*sin(q2) + h2*l2*sin(q2 + q3)*sin(q1)^2*sin(q2) + h2*l2*cos(q2 + q3)*cos(q1)^2*cos(q2) + h2*l2*cos(q2 + q3)*cos(q2)*sin(q1)^2), (l2*sin(q2 + q3) + h2*cos(q2))/(h2*l2*cos(q2 + q3)*cos(q2) + h2*l2*sin(q2 + q3)*sin(q2));
-(l2*cos(q2 + q3)*cos(q2) - l3*sin(q2) + l2*sin(q2 + q3)*sin(q2))/(cos(q1)*(l2*cos(q2 + q3)*cos(q2) + l2*sin(q2 + q3)*sin(q2))),  0,                                    (cos(q1)*sin(q2))/(l2*cos(q2 + q3)*cos(q1)^2*cos(q2) + l2*cos(q2 + q3)*cos(q2)*sin(q1)^2 + l2*sin(q2 + q3)*cos(q1)^2*sin(q2) + l2*sin(q2 + q3)*sin(q1)^2*sin(q2)),                                          (sin(q1)*sin(q2))/(l2*cos(q2 + q3)*cos(q1)^2*cos(q2) + l2*cos(q2 + q3)*cos(q2)*sin(q1)^2 + l2*sin(q2 + q3)*cos(q1)^2*sin(q2) + l2*sin(q2 + q3)*sin(q1)^2*sin(q2)),                             -cos(q2)/(l2*cos(q2 + q3)*cos(q2) + l2*sin(q2 + q3)*sin(q2));
                                                                                                                              0, -1,                                                         -sin(q1)/(l1*sin(q1)^2 + l1*cos(q1)^2 + l2*cos(q2 + q3)*cos(q1)^2 + l2*cos(q2 + q3)*sin(q1)^2 - h2*cos(q1)^2*sin(q2) - h2*sin(q1)^2*sin(q2)),                                                                cos(q1)/(l1*sin(q1)^2 + l1*cos(q1)^2 + l2*cos(q2 + q3)*cos(q1)^2 + l2*cos(q2 + q3)*sin(q1)^2 - h2*cos(q1)^2*sin(q2) - h2*sin(q1)^2*sin(q2)),                                                                                        0]
 
% qvbar = Jv5 \ chi_dot
qv = inv_je * chi_dot
% qv = [qvbar(1); qvbar(2); qvbar(3); -qvbar(2)-qvbar(3); qv5]

end
